simulink model "AEBMIL"  (Simulink 8.2)
settings: Solver=FixedStepDiscrete  StartTime=0.0  StopTime=126  FixedStep=0.005  RelTol=1e-3
PostLoadFcn:
  | , if any(exist('dsrtsu_mdlpostloadfcn', 'file') == [2, 3, 6]), try dsrtsu_mdlpostloadfcn('Execute', bdroot); catch fprintf('Error in PostLoadFcn (dsrtsu_mdlpostloadfcn) for model "%s":\n %s\n', bdroot, lasterr); end, end,
values from neighbouring files (symbols this model uses):
  C_TASK_5MS_S = (	C_TICK_TIME_S      	)    [hcu_local_hdr.m]
  ENUM_GEARPOSN_1ST = uint8(  1  )    [hcu_local_hdr.m]
  ENUM_GEARPOSN_R = uint8(  7  )    [hcu_local_hdr.m]
  FALSE = boolean( 0 )    [hcu_local_hdr.m]
  R_OBJ_Position = single([ii 0 0])    [GridSearch.m]
  R_OBJ_RelAccel = single([0 0 kk])    [GridSearch.m]
  R_OBJ_RelVelocity = single([0 jj 0])    [GridSearch.m]
  TRUE = boolean( 1 )    [hcu_local_hdr.m]
undefined symbols (not defined in the file or in its folder): A_OBJ, AAEB_VehSpd_kph, B_OBJ, C_OBJ, Gamma_OBJ, KAEB_AEBActiveCount_cnt, KAEB_DsblAEBAPPRateThres_pctps, KAEB_DsblAEBSteerRateThres_degps, KAEB_UseMCTTTC_flg, KAEB_VehHoldSpdThres_kph, KOBJ_KalmanFilterCalRate_s, KOBJ_UseCalObjSpd_flg, KOBJ_UseEstObjInfo_flg, KOBJ_VehAccCalRate_s, KOBJ_VehAccFltConst_s, KPTH_ObjPositionYLimit_m, MAEB_AEBTTCThres_s, MAEB_FCWTTCOffset_s, magnitude, MPTH_TurningRadius_m, Q_OBJ, slcm
libraries: simulink x49, hcu_lib x22, dspmtrx3 x3, dspinverses x1
(part 2 of 3)

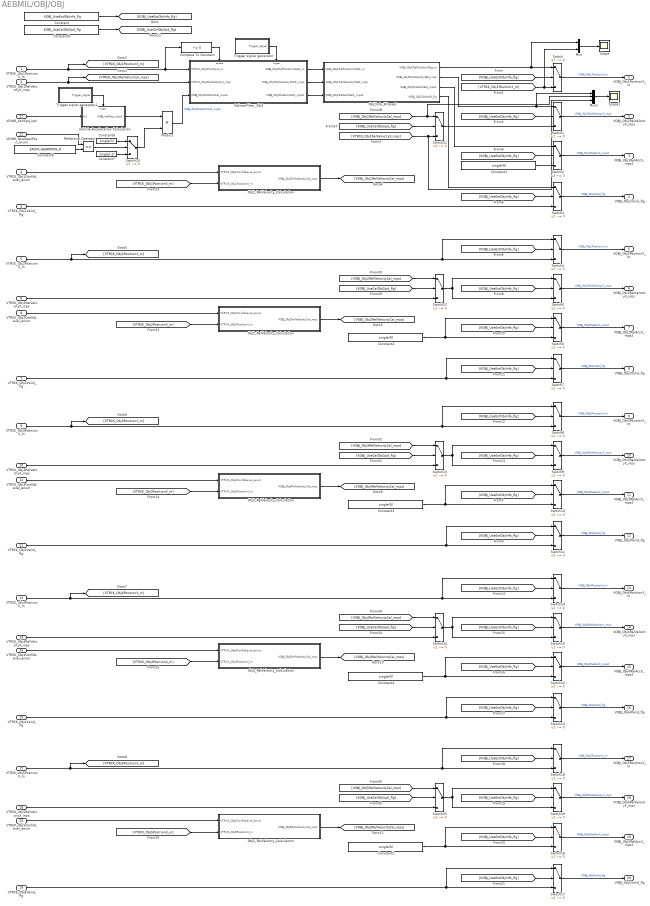
== system AEBMIL/OBJ/OBJ ==
  VTRCK_Obj1PositionX_m : Inport
  VTRCK_Obj1RelVelocityX_mps : Inport  Port=2
  VTRCK_Obj1Valid_flg : Inport  Port=3
  VTRCK_Obj1ConfidLevel_enum : Inport  Port=4
  VTRCK_Obj2PositionX_m : Inport  Port=5
  VTRCK_Obj2RelVelocityX_mps : Inport  Port=6
  VTRCK_Obj2Valid_flg : Inport  Port=7
  VTRCK_Obj2ConfidLevel_enum : Inport  Port=8
  VTRCK_Obj3PositionX_m : Inport  Port=9
  VTRCK_Obj3RelVelocityX_mps : Inport  Port=10
  VTRCK_Obj3Valid_flg : Inport  Port=11
  VTRCK_Obj3ConfidLevel_enum : Inport  Port=12
  VTRCK_Obj4PositionX_m : Inport  Port=13
  VTRCK_Obj4RelVelocityX_mps : Inport  Port=14
  VTRCK_Obj4Valid_flg : Inport  Port=15
  VTRCK_Obj4ConfidLevel_enum : Inport  Port=16
  VTRCK_Obj5PositionX_m : Inport  Port=17
  VTRCK_Obj5RelVelocityX_mps : Inport  Port=18
  VTRCK_Obj5Valid_flg : Inport  Port=19
  VTRCK_Obj5ConfidLevel_enum : Inport  Port=20
  VDINR_VehSpd_kph : Inport  Port=21
  VDINR_NowGearPosn_enum : Inport  Port=22
  Compare To Constant : simulink/Logic and Bit Operations/Compare To Constant  relop=~=  const=0  OutDataTypeStr=boolean
  Constant : Constant  Value=KOBJ_UseEstObjInfo_flg
  Constant{1..5} (5 alike) : Constant  Value=single(0)
  Constant6 : Constant  Value=single(1)
  Constant7 : Constant  Value=single(-1)
  Constant8 : Constant  Value=ENUM_GEARPOSN_R
  Constant9 : Constant  Value=KOBJ_UseCalObjSpd_flg
  KalmanFilter_Obj1 : Subsystem
  Mux : Mux  Inputs=2
  Mux1 : Mux  Inputs=3
  Obj1Info_Filtered : Subsystem
  Obj1_RelVelocity_Calculation : Subsystem
  Obj2_RelVelocity_Calculation : Subsystem
  Obj3_RelVelocity_Calculation : Subsystem
  Obj4_RelVelocity_Calculation : Subsystem
  Obj5_RelVelocity_Calculation : Subsystem
  Product : Product
  Relational Operator : RelationalOperator  Operator===  OutDataTypeStr=boolean
  Scope : Scope
  Scope1 : Scope
  Switch{,1..25} (26 alike) : Switch  Criteria=u2 ~= 0
  Trigger signal generator : Subsystem  TreatAsAtomicUnit=on
  Trigger signal generator1 : Subsystem  TreatAsAtomicUnit=on
  Vehicle Acceleration Calculation : Subsystem
  VOBJ_Obj1PositionX_m : Outport
  VOBJ_Obj1RelVelocityX_mps : Outport  Port=2
  VOBJ_Obj1RelAccX_mps2 : Outport  Port=3
  VOBJ_Obj1Valid_flg : Outport  Port=4
  VOBJ_Obj2PositionX_m : Outport  Port=5
  VOBJ_Obj2RelVelocityX_mps : Outport  Port=6
  VOBJ_Obj2RelAccX_mps2 : Outport  Port=7
  VOBJ_Obj2Valid_flg : Outport  Port=8
  VOBJ_Obj3PositionX_m : Outport  Port=9
  VOBJ_Obj3RelVelocityX_mps : Outport  Port=10
  VOBJ_Obj3RelAccX_mps2 : Outport  Port=11
  VOBJ_Obj3Valid_flg : Outport  Port=12
  VOBJ_Obj4PositionX_m : Outport  Port=13
  VOBJ_Obj4RelVelocityX_mps : Outport  Port=14
  VOBJ_Obj4RelAccX_mps2 : Outport  Port=15
  VOBJ_Obj4Valid_flg : Outport  Port=16
  VOBJ_Obj5PositionX_m : Outport  Port=17
  VOBJ_Obj5RelVelocityX_mps : Outport  Port=18
  VOBJ_Obj5RelAccX_mps2 : Outport  Port=19
  VOBJ_Obj5Valid_flg : Outport  Port=20
  wires:
  Trigger signal generator/1(Trigger_signal) -> KalmanFilter_Obj1/Trigger
  VTRCK_Obj1PositionX_m/1 -> KalmanFilter_Obj1/1(VTRCK_Obj1PositionX_m), Compare To Constant/1, [VTRCK_Obj1PositionX_m]
  VTRCK_Obj1RelVelocityX_mps/1 -> [VTRCK_Obj1RelVelocityX_mps], KalmanFilter_Obj1/2(VTRCK_Obj1RelVelocityX_mps)
  Compare To Constant/1 -> KalmanFilter_Obj1/Enable
  Trigger signal generator1/1(Trigger_signal) -> Vehicle Acceleration Calculation/Trigger
  VDINR_VehSpd_kph/1 -> Vehicle Acceleration Calculation/1(In1)
  Vehicle Acceleration Calculation/1(VOBJ_VehAcc_mps2) -> Product/1
  Product/1 -> KalmanFilter_Obj1/3(VOBJ_Obj1RelAccXCal_mps2)  "VOBJ_Obj1RelAccXCal_mps2"
  KalmanFilter_Obj1/1(VOBJ_Obj1RelPositionXKalF_m) -> Obj1Info_Filtered/1(VOBJ_Obj1RelPositionXKalF_m)
  KalmanFilter_Obj1/2(VOBJ_Obj1RelVelocityXKalF_mps) -> Obj1Info_Filtered/2(VOBJ_Obj1RelVelocityXKalF_mps)
  KalmanFilter_Obj1/3(VOBJ_Obj1RelAccXKalF_mps2) -> Obj1Info_Filtered/3(VOBJ_Obj1RelAccXKalF_mps2)
  VTRCK_Obj1Valid_flg/1 -> Switch3/3
  Constant/1 -> [KOBJ_UseEstObjInfo_flg]
  [KOBJ_UseEstObjInfo_flg] -> Switch/2
  Switch/1 -> VOBJ_Obj1PositionX_m/1  "VOBJ_Obj1PositionX_m"
  [VTRCK_Obj1PositionX_m] -> Mux/2, Switch/3
  Obj1Info_Filtered/1(VOBJ_Obj1RelPositionXEst_m) -> Mux/1, Switch/1
  [KOBJ_UseEstObjInfo_flg] -> Switch1/2
  Switch1/1 -> VOBJ_Obj1RelVelocityX_mps/1  "VOBJ_Obj1RelVelocityX_mps"
  Obj1Info_Filtered/2(VOBJ_Obj1RelVelocityXEst_mps) -> Mux1/1, Switch1/1
  [KOBJ_UseEstObjInfo_flg] -> Switch2/2
  Constant1/1 -> Switch2/3
  Obj1Info_Filtered/3(VOBJ_Obj1RelAccXEst_mps2) -> Switch2/1
  Switch2/1 -> VOBJ_Obj1RelAccX_mps2/1  "VOBJ_Obj1RelAccX_mps2"
  [KOBJ_UseEstObjInfo_flg] -> Switch3/2
  Switch3/1 -> VOBJ_Obj1Valid_flg/1  "VOBJ_Obj1Valid_flg"
  Obj1Info_Filtered/4(VOBJ_Obj1EstValid_flg) -> Switch3/1
  VTRCK_Obj2Valid_flg/1 -> Switch7/1, Switch7/3
  [KOBJ_UseEstObjInfo_flg] -> Switch4/2
  Switch4/1 -> VOBJ_Obj2PositionX_m/1  "VOBJ_Obj2PositionX_m"
  VTRCK_Obj2PositionX_m/1 -> [VTRCK_Obj2PositionX_m], Switch4/1, Switch4/3
  [KOBJ_UseEstObjInfo_flg] -> Switch5/2
  Switch5/1 -> VOBJ_Obj2RelVelocityX_mps/1  "VOBJ_Obj2RelVelocityX_mps"
  [KOBJ_UseEstObjInfo_flg] -> Switch6/2
  Constant2/1 -> Switch6/1, Switch6/3
  Switch6/1 -> VOBJ_Obj2RelAccX_mps2/1  "VOBJ_Obj2RelAccX_mps2"
  [KOBJ_UseEstObjInfo_flg] -> Switch7/2
  Switch7/1 -> VOBJ_Obj2Valid_flg/1  "VOBJ_Obj2Valid_flg"
  VTRCK_Obj3Valid_flg/1 -> Switch11/3, Switch11/1
  [KOBJ_UseEstObjInfo_flg] -> Switch8/2
  Switch8/1 -> VOBJ_Obj3PositionX_m/1  "VOBJ_Obj3PositionX_m"
  VTRCK_Obj3PositionX_m/1 -> [VTRCK_Obj3PositionX_m], Switch8/3, Switch8/1
  [KOBJ_UseEstObjInfo_flg] -> Switch9/2
  Switch9/1 -> VOBJ_Obj3RelVelocityX_mps/1  "VOBJ_Obj3RelVelocityX_mps"
  VTRCK_Obj3RelVelocityX_mps/1 -> Switch23/3
  [KOBJ_UseEstObjInfo_flg] -> Switch10/2
  Constant3/1 -> Switch10/3, Switch10/1
  Switch10/1 -> VOBJ_Obj3RelAccX_mps2/1  "VOBJ_Obj3RelAccX_mps2"
  [KOBJ_UseEstObjInfo_flg] -> Switch11/2
  Switch11/1 -> VOBJ_Obj3Valid_flg/1  "VOBJ_Obj3Valid_flg"
  VTRCK_Obj4Valid_flg/1 -> Switch13/1, Switch13/3
  [KOBJ_UseEstObjInfo_flg] -> Switch14/2
  Switch14/1 -> VOBJ_Obj4PositionX_m/1  "VOBJ_Obj4PositionX_m"
  VTRCK_Obj4PositionX_m/1 -> [VTRCK_Obj4PositionX_m], Switch14/1, Switch14/3
  [KOBJ_UseEstObjInfo_flg] -> Switch15/2
  Switch15/1 -> VOBJ_Obj4RelVelocityX_mps/1  "VOBJ_Obj4RelVelocityX_mps"
  VTRCK_Obj4RelVelocityX_mps/1 -> Switch24/3
  [KOBJ_UseEstObjInfo_flg] -> Switch12/2
  Constant4/1 -> Switch12/1, Switch12/3
  Switch12/1 -> VOBJ_Obj4RelAccX_mps2/1  "VOBJ_Obj4RelAccX_mps2"
  [KOBJ_UseEstObjInfo_flg] -> Switch13/2
  Switch13/1 -> VOBJ_Obj4Valid_flg/1  "VOBJ_Obj4Valid_flg"
  VTRCK_Obj5Valid_flg/1 -> Switch17/3, Switch17/1
  [KOBJ_UseEstObjInfo_flg] -> Switch18/2
  Switch18/1 -> VOBJ_Obj5PositionX_m/1  "VOBJ_Obj5PositionX_m"
  VTRCK_Obj5PositionX_m/1 -> [VTRCK_Obj5PositionX_m], Switch18/3, Switch18/1
  [KOBJ_UseEstObjInfo_flg] -> Switch19/2
  Switch19/1 -> VOBJ_Obj5RelVelocityX_mps/1  "VOBJ_Obj5RelVelocityX_mps"
  VTRCK_Obj5RelVelocityX_mps/1 -> Switch25/3
  [KOBJ_UseEstObjInfo_flg] -> Switch16/2
  Constant5/1 -> Switch16/3, Switch16/1
  Switch16/1 -> VOBJ_Obj5RelAccX_mps2/1  "VOBJ_Obj5RelAccX_mps2"
  [KOBJ_UseEstObjInfo_flg] -> Switch17/2
  Switch17/1 -> VOBJ_Obj5Valid_flg/1  "VOBJ_Obj5Valid_flg"
  VDINR_NowGearPosn_enum/1 -> Relational Operator/1
  Constant8/1 -> Relational Operator/2
  Relational Operator/1 -> Switch20/2
  Constant6/1 -> Switch20/1
  Constant7/1 -> Switch20/3
  Switch20/1 -> Product/2
  VTRCK_Obj5ConfidLevel_enum/1 -> Obj5_RelVelocity_Calculation/1(VTRCK_Obj5ConfidLevel_enum)
  [VTRCK_Obj5PositionX_m] -> Obj5_RelVelocity_Calculation/2(VTRCK_Obj5PositionX_m)
  Obj5_RelVelocity_Calculation/1(VOBJ_Obj5RelVelocityCal_mps) -> [VOBJ_Obj5RelVelocityCal_mps]
  VTRCK_Obj4ConfidLevel_enum/1 -> Obj4_RelVelocity_Calculation/1(VTRCK_Obj4ConfidLevel_enum)
  [VTRCK_Obj4PositionX_m] -> Obj4_RelVelocity_Calculation/2(VTRCK_Obj4PositionX_m)
  Obj4_RelVelocity_Calculation/1(VOBJ_Obj4RelVelocityCal_mps) -> [VOBJ_Obj4RelVelocityCal_mps]
  VTRCK_Obj3ConfidLevel_enum/1 -> Obj3_RelVelocity_Calculation/1(VTRCK_Obj3ConfidLevel_enum)
  [VTRCK_Obj3PositionX_m] -> Obj3_RelVelocity_Calculation/2(VTRCK_Obj3PositionX_m)
  Obj3_RelVelocity_Calculation/1(VOBJ_Obj3RelVelocityCal_mps) -> [VOBJ_Obj3RelVelocityCal_mps]
  VTRCK_Obj2ConfidLevel_enum/1 -> Obj2_RelVelocity_Calculation/1(VTRCK_Obj2ConfidLevel_enum)
  [VTRCK_Obj2PositionX_m] -> Obj2_RelVelocity_Calculation/2(VTRCK_Obj2PositionX_m)
  Obj2_RelVelocity_Calculation/1(VOBJ_Obj2RelVelocityCal_mps) -> [VOBJ_Obj2RelVelocityCal_mps]
  VTRCK_Obj1ConfidLevel_enum/1 -> Obj1_RelVelocity_Calculation/1(VTRCK_Obj1ConfidLevel_enum)
  [VTRCK_Obj1PositionX_m] -> Obj1_RelVelocity_Calculation/2(VTRCK_Obj1PositionX_m)
  Obj1_RelVelocity_Calculation/1(VOBJ_Obj1RelVelocityCal_mps) -> [VOBJ_Obj1RelVelocityCal_mps]
  Constant9/1 -> [KOBJ_UseCalObjSpd_flg]
  [KOBJ_UseCalObjSpd_flg] -> Switch21/2
  [VOBJ_Obj1RelVelocityCal_mps] -> Mux1/2, Switch21/1
  [VTRCK_Obj1RelVelocityX_mps] -> Mux1/3, Switch21/3
  Switch21/1 -> Switch1/3
  [KOBJ_UseCalObjSpd_flg] -> Switch22/2
  [VOBJ_Obj2RelVelocityCal_mps] -> Switch22/1
  VTRCK_Obj2RelVelocityX_mps/1 -> Switch22/3
  Switch22/1 -> Switch5/3, Switch5/1
  [KOBJ_UseCalObjSpd_flg] -> Switch23/2
  [VOBJ_Obj3RelVelocityCal_mps] -> Switch23/1
  Switch23/1 -> Switch9/1, Switch9/3
  [KOBJ_UseCalObjSpd_flg] -> Switch24/2
  [VOBJ_Obj4RelVelocityCal_mps] -> Switch24/1
  Switch24/1 -> Switch15/1, Switch15/3
  [KOBJ_UseCalObjSpd_flg] -> Switch25/2
  [VOBJ_Obj5RelVelocityCal_mps] -> Switch25/1
  Switch25/1 -> Switch19/1, Switch19/3
  Mux/1 -> Scope/1
  Mux1/1 -> Scope1/1

== system AEBMIL/OBJ/model_info ==
  EmptySubsystem : Subsystem

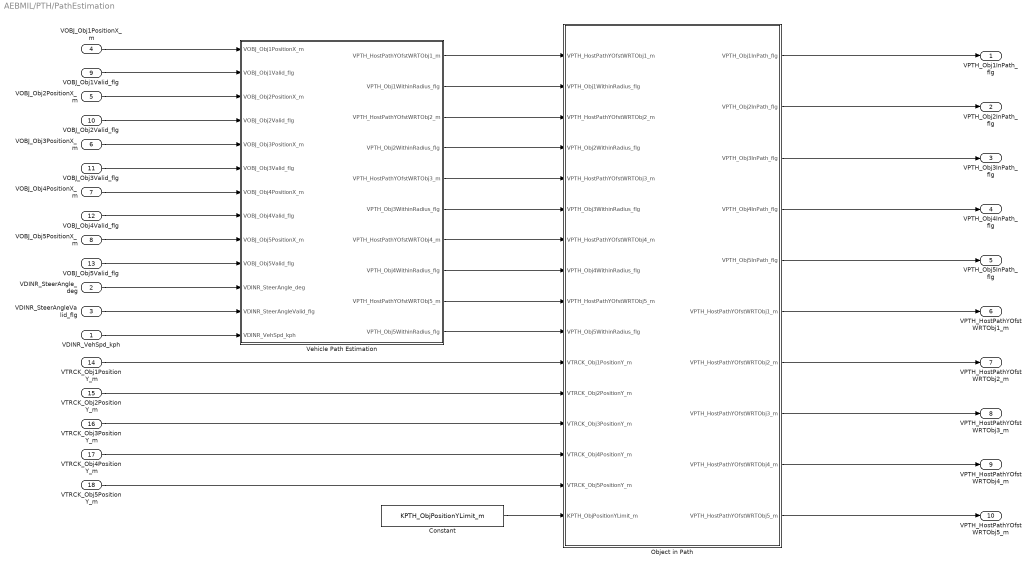
== system AEBMIL/PTH/PathEstimation ==
  VDINR_VehSpd_kph : Inport
  VDINR_SteerAngle_deg : Inport  Port=2
  VDINR_SteerAngleValid_flg : Inport  Port=3
  VOBJ_Obj1PositionX_m : Inport  Port=4
  VOBJ_Obj2PositionX_m : Inport  Port=5
  VOBJ_Obj3PositionX_m : Inport  Port=6
  VOBJ_Obj4PositionX_m : Inport  Port=7
  VOBJ_Obj5PositionX_m : Inport  Port=8
  VOBJ_Obj1Valid_flg : Inport  Port=9
  VOBJ_Obj2Valid_flg : Inport  Port=10
  VOBJ_Obj3Valid_flg : Inport  Port=11
  VOBJ_Obj4Valid_flg : Inport  Port=12
  VOBJ_Obj5Valid_flg : Inport  Port=13
  VTRCK_Obj1PositionY_m : Inport  Port=14
  VTRCK_Obj2PositionY_m : Inport  Port=15
  VTRCK_Obj3PositionY_m : Inport  Port=16
  VTRCK_Obj4PositionY_m : Inport  Port=17
  VTRCK_Obj5PositionY_m : Inport  Port=18
  Constant : Constant  Value=KPTH_ObjPositionYLimit_m
  Object in Path : Subsystem
  Vehicle Path Estimation : Subsystem
  VPTH_Obj1InPath_flg : Outport
  VPTH_Obj2InPath_flg : Outport  Port=2
  VPTH_Obj3InPath_flg : Outport  Port=3
  VPTH_Obj4InPath_flg : Outport  Port=4
  VPTH_Obj5InPath_flg : Outport  Port=5
  VPTH_HostPathYOfstWRTObj1_m : Outport  Port=6
  VPTH_HostPathYOfstWRTObj2_m : Outport  Port=7
  VPTH_HostPathYOfstWRTObj3_m : Outport  Port=8
  VPTH_HostPathYOfstWRTObj4_m : Outport  Port=9
  VPTH_HostPathYOfstWRTObj5_m : Outport  Port=10
  wires:
  Object in Path/10("VPTH_HostPathYOfstWRTObj5_m ") -> VPTH_HostPathYOfstWRTObj5_m/1
  Object in Path/9("VPTH_HostPathYOfstWRTObj4_m ") -> VPTH_HostPathYOfstWRTObj4_m/1
  Object in Path/8("VPTH_HostPathYOfstWRTObj3_m ") -> VPTH_HostPathYOfstWRTObj3_m/1
  Object in Path/7("VPTH_HostPathYOfstWRTObj2_m ") -> VPTH_HostPathYOfstWRTObj2_m/1
  Object in Path/6("VPTH_HostPathYOfstWRTObj1_m ") -> VPTH_HostPathYOfstWRTObj1_m/1
  VOBJ_Obj5Valid_flg/1 -> Vehicle Path Estimation/10(VOBJ_Obj5Valid_flg)
  VOBJ_Obj4Valid_flg/1 -> Vehicle Path Estimation/8(VOBJ_Obj4Valid_flg)
  VOBJ_Obj3Valid_flg/1 -> Vehicle Path Estimation/6(VOBJ_Obj3Valid_flg)
  VOBJ_Obj2Valid_flg/1 -> Vehicle Path Estimation/4(VOBJ_Obj2Valid_flg)
  VOBJ_Obj1Valid_flg/1 -> Vehicle Path Estimation/2(VOBJ_Obj1Valid_flg)
  Object in Path/5(VPTH_Obj5InPath_flg) -> VPTH_Obj5InPath_flg/1
  Object in Path/4(VPTH_Obj4InPath_flg) -> VPTH_Obj4InPath_flg/1
  Object in Path/3(VPTH_Obj3InPath_flg) -> VPTH_Obj3InPath_flg/1
  Object in Path/2(VPTH_Obj2InPath_flg) -> VPTH_Obj2InPath_flg/1
  VTRCK_Obj2PositionY_m/1 -> Object in Path/12(VTRCK_Obj2PositionY_m)
  VTRCK_Obj3PositionY_m/1 -> Object in Path/13(VTRCK_Obj3PositionY_m)
  VTRCK_Obj5PositionY_m/1 -> Object in Path/15(VTRCK_Obj5PositionY_m)
  VTRCK_Obj4PositionY_m/1 -> Object in Path/14(VTRCK_Obj4PositionY_m)
  Vehicle Path Estimation/10(VPTH_Obj5WithinRadius_flg) -> Object in Path/10(VPTH_Obj5WithinRadius_flg)
  Vehicle Path Estimation/9(VPTH_HostPathYOfstWRTObj5_m) -> Object in Path/9(VPTH_HostPathYOfstWRTObj5_m)
  Vehicle Path Estimation/8(VPTH_Obj4WithinRadius_flg) -> Object in Path/8(VPTH_Obj4WithinRadius_flg)
  Vehicle Path Estimation/7(VPTH_HostPathYOfstWRTObj4_m) -> Object in Path/7(VPTH_HostPathYOfstWRTObj4_m)
  Vehicle Path Estimation/6(VPTH_Obj3WithinRadius_flg) -> Object in Path/6(VPTH_Obj3WithinRadius_flg)
  Vehicle Path Estimation/5(VPTH_HostPathYOfstWRTObj3_m) -> Object in Path/5(VPTH_HostPathYOfstWRTObj3_m)
  Vehicle Path Estimation/4(VPTH_Obj2WithinRadius_flg) -> Object in Path/4(VPTH_Obj2WithinRadius_flg)
  Vehicle Path Estimation/3(VPTH_HostPathYOfstWRTObj2_m) -> Object in Path/3(VPTH_HostPathYOfstWRTObj2_m)
  VOBJ_Obj5PositionX_m/1 -> Vehicle Path Estimation/9(VOBJ_Obj5PositionX_m)
  VOBJ_Obj4PositionX_m/1 -> Vehicle Path Estimation/7(VOBJ_Obj4PositionX_m)
  VOBJ_Obj3PositionX_m/1 -> Vehicle Path Estimation/5(VOBJ_Obj3PositionX_m)
  VOBJ_Obj2PositionX_m/1 -> Vehicle Path Estimation/3(VOBJ_Obj2PositionX_m)
  VDINR_SteerAngleValid_flg/1 -> Vehicle Path Estimation/12(VDINR_SteerAngleValid_flg)
  VDINR_VehSpd_kph/1 -> Vehicle Path Estimation/13(VDINR_VehSpd_kph)
  VOBJ_Obj1PositionX_m/1 -> Vehicle Path Estimation/1(VOBJ_Obj1PositionX_m)
  VDINR_SteerAngle_deg/1 -> Vehicle Path Estimation/11(VDINR_SteerAngle_deg)
  VTRCK_Obj1PositionY_m/1 -> Object in Path/11(VTRCK_Obj1PositionY_m)
  Constant/1 -> Object in Path/16(KPTH_ObjPositionYLimit_m)
  Vehicle Path Estimation/1(VPTH_HostPathYOfstWRTObj1_m) -> Object in Path/1(VPTH_HostPathYOfstWRTObj1_m)
  Object in Path/1(VPTH_Obj1InPath_flg) -> VPTH_Obj1InPath_flg/1
  Vehicle Path Estimation/2(VPTH_Obj1WithinRadius_flg) -> Object in Path/2(VPTH_Obj1WithinRadius_flg)

== system AEBMIL/PTH/model_info ==
  EmptySubsystem : Subsystem

== system AEBMIL/TTC/MCT_TTC_Calculation ==
  VMCT_MCTRelPositionX_m : Inport
  VMCT_MCTRelVelocityX_mps : Inport  Port=2
  VMCT_MCTValid_flg : Inport  Port=3
  VMCT_MCTInPath_flg : Inport  Port=4
  Constant1 : Constant  Value=-99  OutDataTypeStr=single
  Data Type Conversion : DataTypeConversion  OutDataTypeStr=single
  Data Type Conversion1 : DataTypeConversion  OutDataTypeStr=single
  Gain4 : Gain  Gain=-1
  Product : Product  Inputs=3  RndMeth=Zero
  divide : hcu_lib/divide
  VTTC_MCTTTC_s : Outport
  wires:
  Data Type Conversion1/1 -> Product/3
  Data Type Conversion/1 -> Product/2
  VMCT_MCTInPath_flg/1 -> Data Type Conversion1/1
  VMCT_MCTRelVelocityX_mps/1 -> Product/1
  VMCT_MCTRelPositionX_m/1 -> divide/1
  Product/1 -> divide/2
  VMCT_MCTValid_flg/1 -> Data Type Conversion/1
  Constant1/1 -> divide/3
  divide/1 -> Gain4/1
  Gain4/1 -> VTTC_MCTTTC_s/1  "VTTC_MCTTTC_s"

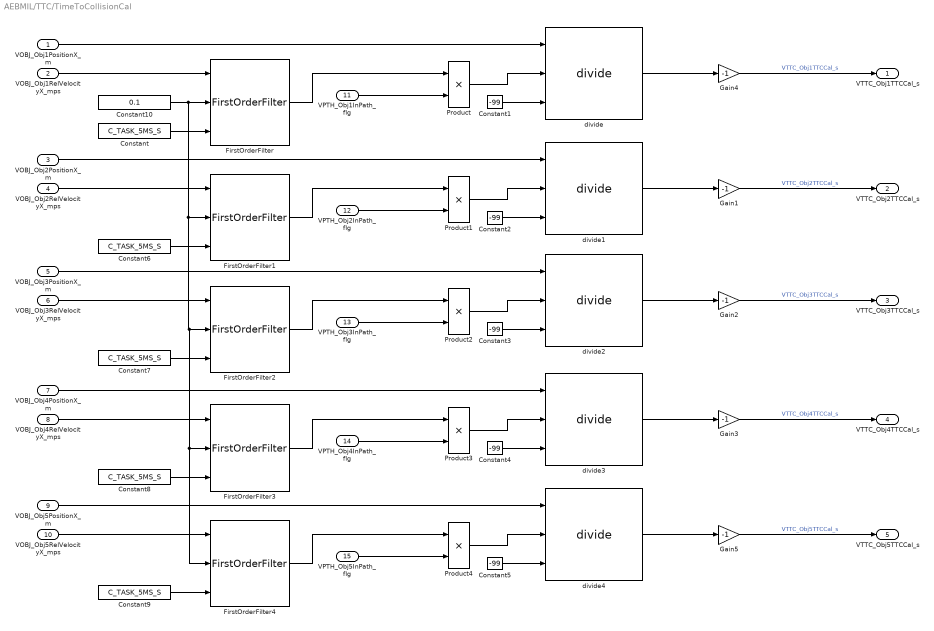
== system AEBMIL/TTC/TimeToCollisionCal ==
  VOBJ_Obj1PositionX_m : Inport
  VOBJ_Obj1RelVelocityX_mps : Inport  Port=2
  VOBJ_Obj2PositionX_m : Inport  Port=3
  VOBJ_Obj2RelVelocityX_mps : Inport  Port=4
  VOBJ_Obj3PositionX_m : Inport  Port=5
  VOBJ_Obj3RelVelocityX_mps : Inport  Port=6
  VOBJ_Obj4PositionX_m : Inport  Port=7
  VOBJ_Obj4RelVelocityX_mps : Inport  Port=8
  VOBJ_Obj5PositionX_m : Inport  Port=9
  VOBJ_Obj5RelVelocityX_mps : Inport  Port=10
  VPTH_Obj1InPath_flg : Inport  Port=11
  VPTH_Obj2InPath_flg : Inport  Port=12
  VPTH_Obj3InPath_flg : Inport  Port=13
  VPTH_Obj4InPath_flg : Inport  Port=14
  VPTH_Obj5InPath_flg : Inport  Port=15
  Constant{,6..9} (5 alike) : Constant  Value=C_TASK_5MS_S
  Constant{1..5} (5 alike) : Constant  Value=-99  OutDataTypeStr=single
  Constant10 : Constant  Value=0.1  OutDataTypeStr=single
  FirstOrderFilter{,1..4} (5 alike) : hcu_lib/FirstOrderFilter
  Gain{1..5} (5 alike) : Gain  Gain=-1
  Product{,1..4} (5 alike) : Product  RndMeth=Zero
  divide{,1..4} (5 alike) : hcu_lib/divide
  VTTC_Obj1TTCCal_s : Outport
  VTTC_Obj2TTCCal_s : Outport  Port=2
  VTTC_Obj3TTCCal_s : Outport  Port=3
  VTTC_Obj4TTCCal_s : Outport  Port=4
  VTTC_Obj5TTCCal_s : Outport  Port=5
  wires:
  FirstOrderFilter4/1 -> Product4/1
  FirstOrderFilter3/1 -> Product3/1
  FirstOrderFilter2/1 -> Product2/1
  FirstOrderFilter1/1 -> Product1/1
  FirstOrderFilter/1 -> Product/1
  divide4/1 -> Gain5/1
  divide3/1 -> Gain3/1
  divide2/1 -> Gain2/1
  divide1/1 -> Gain1/1
  divide/1 -> Gain4/1
  Constant10/1 -> FirstOrderFilter/2, FirstOrderFilter1/2, FirstOrderFilter2/2, FirstOrderFilter3/2, FirstOrderFilter4/2
  Constant9/1 -> FirstOrderFilter4/3
  Constant8/1 -> FirstOrderFilter3/3
  Constant7/1 -> FirstOrderFilter2/3
  Constant6/1 -> FirstOrderFilter1/3
  Constant/1 -> FirstOrderFilter/3
  VOBJ_Obj5PositionX_m/1 -> divide4/1
  Gain5/1 -> VTTC_Obj5TTCCal_s/1  "VTTC_Obj5TTCCal_s"
  VOBJ_Obj5RelVelocityX_mps/1 -> FirstOrderFilter4/1
  Constant5/1 -> divide4/3
  VPTH_Obj5InPath_flg/1 -> Product4/2
  Product4/1 -> divide4/2
  VOBJ_Obj4PositionX_m/1 -> divide3/1
  Gain3/1 -> VTTC_Obj4TTCCal_s/1  "VTTC_Obj4TTCCal_s"
  VOBJ_Obj4RelVelocityX_mps/1 -> FirstOrderFilter3/1
  Constant4/1 -> divide3/3
  VPTH_Obj4InPath_flg/1 -> Product3/2
  Product3/1 -> divide3/2
  VOBJ_Obj3PositionX_m/1 -> divide2/1
  Gain2/1 -> VTTC_Obj3TTCCal_s/1  "VTTC_Obj3TTCCal_s"
  VOBJ_Obj3RelVelocityX_mps/1 -> FirstOrderFilter2/1
  Constant3/1 -> divide2/3
  VPTH_Obj3InPath_flg/1 -> Product2/2
  Product2/1 -> divide2/2
  VOBJ_Obj2PositionX_m/1 -> divide1/1
  Gain1/1 -> VTTC_Obj2TTCCal_s/1  "VTTC_Obj2TTCCal_s"
  VOBJ_Obj2RelVelocityX_mps/1 -> FirstOrderFilter1/1
  Constant2/1 -> divide1/3
  VPTH_Obj2InPath_flg/1 -> Product1/2
  Product1/1 -> divide1/2
  VOBJ_Obj1PositionX_m/1 -> divide/1
  Gain4/1 -> VTTC_Obj1TTCCal_s/1  "VTTC_Obj1TTCCal_s"
  VOBJ_Obj1RelVelocityX_mps/1 -> FirstOrderFilter/1
  Constant1/1 -> divide/3
  VPTH_Obj1InPath_flg/1 -> Product/2
  Product/1 -> divide/2

== system AEBMIL/TTC/model_info ==
  EmptySubsystem : Subsystem

== system AEBMIL/AEB/AEB/AEB Determination ==
  VAEB_DriverDisable_flg : Inport
  VAEB_DriverDisableLatch_flg : Inport  Port=2
  VDINR_SeatBeltNOTFasten_flg : Inport  Port=3
  VDINR_VehSpd_kph : Inport  Port=4
  VTTC_MCTTTC_s : Inport  Port=5
  VTTC_Obj1TTCCal_s : Inport  Port=6
  AEB_Brain : Subsystem
  LookAhead Distance Gain Lookup1 : Lookup  InputValues=AAEB_VehSpd_kph  Table=MAEB_FCWTTCOffset_s  LookUpMeth=Interpolation-Use End Values
      settings: AttributesFormatString=%<InputValues>\n%<Table>
  LookAhead Distance Gain Lookup2 : Lookup  InputValues=AAEB_VehSpd_kph  Table=MAEB_AEBTTCThres_s  LookUpMeth=Interpolation-Use End Values
      settings: AttributesFormatString=%<InputValues>\n%<Table>
  Terminator : Terminator
  VAEB_AEBActive_flg : Outport
  VAEB_FCWActive_flg : Outport  Port=2
  VAEB_ForcedIdle_flg : Outport  Port=3
  VAEB_PreFillReq_flg : Outport  Port=4
  VAEB_VehHoldReq_flg : Outport  Port=5
  wires:
  VTTC_Obj1TTCCal_s/1 -> AEB_Brain/7(VTTC_Obj1TTCCal_s)
  AEB_Brain/5(VAEB_VehHoldReq_flg) -> VAEB_VehHoldReq_flg/1
  AEB_Brain/4(VAEB_PreFillReq_flg) -> VAEB_PreFillReq_flg/1
  AEB_Brain/3(VAEB_ForcedIdle_flg) -> VAEB_ForcedIdle_flg/1
  AEB_Brain/2(VAEB_FCWActive_flg) -> VAEB_FCWActive_flg/1
  VTTC_MCTTTC_s/1 -> AEB_Brain/6(VTTC_MCTTTC_s)
  VDINR_SeatBeltNOTFasten_flg/1 -> AEB_Brain/5(VDINR_SeatBeltNOTFasten_flg)
  VAEB_DriverDisableLatch_flg/1 -> Terminator/1
  LookAhead Distance Gain Lookup1/1 -> AEB_Brain/2(FCWTTCOffset)
  AEB_Brain/1(VAEB_AEBActive_flg) -> VAEB_AEBActive_flg/1
  VDINR_VehSpd_kph/1 -> LookAhead Distance Gain Lookup2/1, LookAhead Distance Gain Lookup1/1, AEB_Brain/3(VDINR_VehSpd_kph)
  LookAhead Distance Gain Lookup2/1 -> AEB_Brain/1(AEBTTCThres)
  VAEB_DriverDisable_flg/1 -> AEB_Brain/4(VAEB_DriverDisable_flg)

== system AEBMIL/AEB/AEB/Driver Disable ==
  VDINR_SteerAngle_deg : Inport
  VDINR_SteerAngleValid_flg : Inport  Port=2
  VDINR_HWAccelPedalPosn_pct : Inport  Port=3
  VDINR_HWAccelPedalPosnValid_flg : Inport  Port=4
  VAEB_AEBActive_flg : Inport  Port=5
  APPRateCalculation : Subsystem  TreatAsAtomicUnit=on
  Abs1 : Abs
  Constant1 : Constant  Value=KAEB_DsblAEBAPPRateThres_pctps
  Constant2 : Constant  Value=KAEB_DsblAEBSteerRateThres_degps
  Function-Call Generator : Stateflow chart  TreatAsAtomicUnit=on
  Logical Operator : Logic  Operator=NOT  AllPortsSameDT=off  OutDataTypeStr=boolean
  Logical Operator8 : Logic  Operator=OR  AllPortsSameDT=off  OutDataTypeStr=boolean
  Relational Operator1 : RelationalOperator  OutDataTypeStr=boolean
  Relational Operator3 : RelationalOperator  OutDataTypeStr=boolean
  SR-Latch : hcu_lib/SR-Latch
  SteeringRateCalculation : Subsystem  TreatAsAtomicUnit=on
  VAEB_DriverDisable_flg : Outport
  VAEB_DriverDisableLatch_flg : Outport  Port=2
  wires:
  Logical Operator/1 -> SR-Latch/2
  SR-Latch/1 -> VAEB_DriverDisableLatch_flg/1  "VAEB_DriverDisableLatch_flg"
  Logical Operator8/1 -> SR-Latch/1, VAEB_DriverDisable_flg/1  "VAEB_DriverDisable_flg"
  VAEB_AEBActive_flg/1 -> Logical Operator/1
  Relational Operator1/1 -> Logical Operator8/2
  APPRateCalculation/1(VAEB_APPMovingRate_pctps) -> Relational Operator1/1
  Abs1/1 -> Relational Operator3/1
  Constant1/1 -> Relational Operator1/2
  VDINR_HWAccelPedalPosnValid_flg/1 -> APPRateCalculation/2(VDINR_HWAccelPedalPosnValid_flg)
  VDINR_HWAccelPedalPosn_pct/1 -> APPRateCalculation/1(VDINR_HWAccelPedalPosn_pct)
  SteeringRateCalculation/1(VAEB_SteeringRate_degps) -> Abs1/1
  VDINR_SteerAngleValid_flg/1 -> SteeringRateCalculation/2(VDINR_SteerAngleValid_flg)
  [trig_APPINTEND] -> APPRateCalculation/Trigger
  [trig_STEERINTEND] -> SteeringRateCalculation/Trigger
  Function-Call Generator/2(trig_APPINTEND()) -> [trig_APPINTEND]
  Function-Call Generator/1(trig_STEERINTEND()) -> [trig_STEERINTEND]
  VDINR_SteerAngle_deg/1 -> SteeringRateCalculation/1(VDINR_SteerAngle_deg)
  Relational Operator3/1 -> Logical Operator8/1
  Constant2/1 -> Relational Operator3/2

== system AEBMIL/AEB/model_info/EmptySubsystem ==

== system AEBMIL/MCT/MCT/Switch Case Action Subsystem ==
  Action Port : ActionPort  ActionType=then
  Constant : Constant  Value=uint8(1)
  Out1 : Outport
  wires:
  Constant/1 -> Out1/1

== system AEBMIL/MCT/MCT/Switch Case Action Subsystem1 ==
  Action Port : ActionPort  ActionType=elseif
  Constant : Constant  Value=uint8(2)
  Out1 : Outport
  wires:
  Constant/1 -> Out1/1

== system AEBMIL/MCT/MCT/Switch Case Action Subsystem2 ==
  Action Port : ActionPort  ActionType=elseif
  Constant : Constant  Value=uint8(3)
  Out1 : Outport
  wires:
  Constant/1 -> Out1/1

== system AEBMIL/MCT/MCT/Switch Case Action Subsystem3 ==
  Action Port : ActionPort  ActionType=elseif
  Constant : Constant  Value=uint8(4)
  Out1 : Outport
  wires:
  Constant/1 -> Out1/1

== system AEBMIL/MCT/MCT/Switch Case Action Subsystem4 ==
  Action Port : ActionPort  ActionType=elseif
  Constant : Constant  Value=uint8(5)
  Out1 : Outport
  wires:
  Constant/1 -> Out1/1

== system AEBMIL/MCT/MCT/Switch Case Action Subsystem5 ==
  Action Port : ActionPort  ActionType=else
  Constant : Constant  Value=uint8(0)
  Out1 : Outport
  wires:
  Constant/1 -> Out1/1

== system AEBMIL/MCT/model_info/EmptySubsystem ==

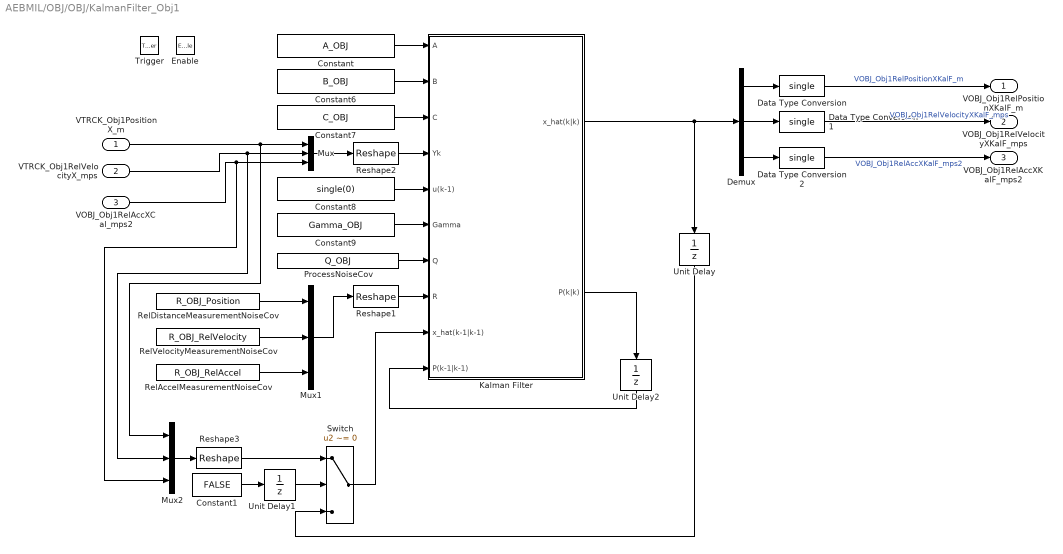
== system AEBMIL/OBJ/OBJ/KalmanFilter_Obj1 ==
  VTRCK_Obj1PositionX_m : Inport
  VTRCK_Obj1RelVelocityX_mps : Inport  Port=2
  VOBJ_Obj1RelAccXCal_mps2 : Inport  Port=3
  Enable : EnablePort  StatesWhenEnabling=reset
  Trigger : TriggerPort  PortDimensions=1
  Constant : Constant  Value=A_OBJ
  Constant1 : Constant  Value=FALSE
  Constant6 : Constant  Value=B_OBJ
  Constant7 : Constant  Value=C_OBJ
  Constant8 : Constant  Value=single(0)
  Constant9 : Constant  Value=Gamma_OBJ
  Data Type Conversion : DataTypeConversion  OutDataTypeStr=single
  Data Type Conversion1 : DataTypeConversion  OutDataTypeStr=single
  Data Type Conversion2 : DataTypeConversion  OutDataTypeStr=single
  Demux : Demux  Outputs=3
  Kalman Filter : Subsystem
  Mux : Mux  Inputs=3
  Mux1 : Mux  Inputs=3
  Mux2 : Mux  Inputs=3
  ProcessNoiseCov : Constant  Value=Q_OBJ
  RelAccelMeasurementNoiseCov : Constant  Value=R_OBJ_RelAccel  OutDataTypeStr=single
  RelDistanceMeasurementNoiseCov : Constant  Value=R_OBJ_Position  OutDataTypeStr=single
  RelVelocityMeasurementNoiseCov : Constant  Value=R_OBJ_RelVelocity  OutDataTypeStr=single
  Reshape1 : Reshape  OutputDimensionality=Customize  OutputDimensions=[3,3]
  Reshape2 : Reshape  OutputDimensionality=Customize  OutputDimensions=[3,1]
  Reshape3 : Reshape  OutputDimensionality=Customize  OutputDimensions=[3,1]
  Switch : Switch  Criteria=u2 ~= 0
  Unit Delay : UnitDelay  InitialCondition=single([0;0;0])  SampleTime=-1
  Unit Delay1 : UnitDelay  InitialCondition=TRUE  SampleTime=-1
  Unit Delay2 : UnitDelay  InitialCondition=single(eye(3,3))  SampleTime=-1
  VOBJ_Obj1RelPositionXKalF_m : Outport  OutputWhenDisabled=reset  InitialOutput=[0]
  VOBJ_Obj1RelVelocityXKalF_mps : Outport  Port=2  OutputWhenDisabled=reset  InitialOutput=[0]
  VOBJ_Obj1RelAccXKalF_mps2 : Outport  Port=3  OutputWhenDisabled=reset  InitialOutput=[0]
  wires:
  Data Type Conversion2/1 -> VOBJ_Obj1RelAccXKalF_mps2/1  "VOBJ_Obj1RelAccXKalF_mps2"
  Data Type Conversion1/1 -> VOBJ_Obj1RelVelocityXKalF_mps/1  "VOBJ_Obj1RelVelocityXKalF_mps"
  Data Type Conversion/1 -> VOBJ_Obj1RelPositionXKalF_m/1  "VOBJ_Obj1RelPositionXKalF_m"
  Kalman Filter/2(P(k|k)) -> Unit Delay2/1
  Unit Delay2/1 -> Kalman Filter/10(P(k-1|k-1))
  Kalman Filter/1(x_hat(k|k)) -> Unit Delay/1, Demux/1
  Unit Delay/1 -> Switch/3
  Constant9/1 -> Kalman Filter/6(Gamma)
  ProcessNoiseCov/1 -> Kalman Filter/7(Q)
  Mux1/1 -> Reshape1/1
  Reshape2/1 -> Kalman Filter/4(Yk)
  Mux/1 -> Reshape2/1
  Constant8/1 -> Kalman Filter/5(u(k-1))
  Constant/1 -> Kalman Filter/1(A)
  Constant6/1 -> Kalman Filter/2(B)
  Constant7/1 -> Kalman Filter/3(C)
  RelDistanceMeasurementNoiseCov/1 -> Mux1/1
  RelVelocityMeasurementNoiseCov/1 -> Mux1/2
  Reshape1/1 -> Kalman Filter/8(R)
  VTRCK_Obj1RelVelocityX_mps/1 -> Mux2/2, Mux/2
  VTRCK_Obj1PositionX_m/1 -> Mux2/1, Mux/1
  Demux/2 -> Data Type Conversion1/1
  Demux/1 -> Data Type Conversion/1
  Demux/3 -> Data Type Conversion2/1
  Constant1/1 -> Unit Delay1/1
  Unit Delay1/1 -> Switch/2
  VOBJ_Obj1RelAccXCal_mps2/1 -> Mux2/3, Mux/3
  Mux2/1 -> Reshape3/1
  Reshape3/1 -> Switch/1
  Switch/1 -> Kalman Filter/9(x_hat(k-1|k-1))
  RelAccelMeasurementNoiseCov/1 -> Mux1/3

== system AEBMIL/OBJ/OBJ/Obj1Info_Filtered ==
  VOBJ_Obj1RelPositionXKalF_m : Inport
  VOBJ_Obj1RelVelocityXKalF_mps : Inport  Port=2
  VOBJ_Obj1RelAccXKalF_mps2 : Inport  Port=3
  Compare To Zero : simulink/Logic and Bit Operations/Compare To Zero  relop=~=  OutDataTypeStr=boolean
  Constant : Constant  Value=single(0)
  Constant1 : Constant  Value=single(0)
  Constant2 : Constant  Value=single(0)
  Switch : Switch  Criteria=u2 ~= 0
  Switch1 : Switch  Criteria=u2 ~= 0
  Switch2 : Switch  Criteria=u2 ~= 0
  VOBJ_Obj1RelPositionXEst_m : Outport
  VOBJ_Obj1RelVelocityXEst_mps : Outport  Port=2
  VOBJ_Obj1RelAccXEst_mps2 : Outport  Port=3
  VOBJ_Obj1EstValid_flg : Outport  Port=4
  wires:
  VOBJ_Obj1RelPositionXKalF_m/1 -> Switch/1, Compare To Zero/1
  Compare To Zero/1 -> [VOBJ_Obj1EstValid_flg]
  [VOBJ_Obj1EstValid_flg] -> VOBJ_Obj1EstValid_flg/1  "VOBJ_Obj1EstValid_flg"
  [VOBJ_Obj1EstValid_flg] -> Switch/2
  Switch/1 -> VOBJ_Obj1RelPositionXEst_m/1  "VOBJ_Obj1RelPositionXEst_m"
  Constant/1 -> Switch/3
  [VOBJ_Obj1EstValid_flg] -> Switch1/2
  Switch1/1 -> VOBJ_Obj1RelVelocityXEst_mps/1  "VOBJ_Obj1RelVelocityXEst_mps"
  Constant1/1 -> Switch1/3
  [VOBJ_Obj1EstValid_flg] -> Switch2/2
  Switch2/1 -> VOBJ_Obj1RelAccXEst_mps2/1  "VOBJ_Obj1RelAccXEst_mps2"
  Constant2/1 -> Switch2/3
  VOBJ_Obj1RelVelocityXKalF_mps/1 -> Switch1/1
  VOBJ_Obj1RelAccXKalF_mps2/1 -> Switch2/1

== system AEBMIL/OBJ/OBJ/Obj1_RelVelocity_Calculation ==
  VTRCK_Obj1ConfidLevel_enum : Inport
  VTRCK_Obj1PositionX_m : Inport  Port=2
  Compare To Constant2 : simulink/Logic and Bit Operations/Compare To Constant  relop=~=  const=0  OutDataTypeStr=boolean
  DataPass_Obj1 : Subsystem  TreatAsAtomicUnit=on
  Detect Change1 : simulink/Logic and Bit Operations/Detect Change  vinit=0  InputProcessing=Inherited  OutDataTypeStr=boolean
  Detect Decrease : simulink/Logic and Bit Operations/Detect Decrease  vinit=0.0  InputProcessing=Inherited  OutDataTypeStr=boolean
  Detect Increase : simulink/Logic and Bit Operations/Detect Increase  vinit=0.0  InputProcessing=Inherited  OutDataTypeStr=boolean
  Logical Operator3 : Logic  Operator=NOT  AllPortsSameDT=off  OutDataTypeStr=boolean
  Logical Operator4 : Logic  AllPortsSameDT=off  OutDataTypeStr=boolean
  Obj1_RelVelocity_Cal : Subsystem
  SR-Latch : hcu_lib/SR-Latch
  SandH_Obj1 : Subsystem  TreatAsAtomicUnit=on
  Timer1 : Subsystem  TreatAsAtomicUnit=on
  Unit Delay1 : UnitDelay  SampleTime=-1
  VOBJ_Obj1RelVelocityCal_mps : Outport
  wires:
  Obj1_RelVelocity_Cal/1(VOBJ_Obj1RelVelocityCal_mps) -> VOBJ_Obj1RelVelocityCal_mps/1
  Compare To Constant2/1 -> Logical Operator4/2
  Unit Delay1/1 -> Logical Operator3/1
  Logical Operator4/1 -> Timer1/Enable
  Logical Operator3/1 -> Logical Operator4/1
  SandH_Obj1/1(Out1) -> Obj1_RelVelocity_Cal/2(TimeDur_s)
  Timer1/1(Timer (sec)) -> SandH_Obj1/1(In1)
  DataPass_Obj1/1(Out1) -> Obj1_RelVelocity_Cal/1(ObjPositionX_m), Detect Change1/1, Compare To Constant2/1
  Detect Change1/1 -> Unit Delay1/1, SandH_Obj1/Trigger, Obj1_RelVelocity_Cal/Trigger
  VTRCK_Obj1PositionX_m/1 -> DataPass_Obj1/1(In1)
  SR-Latch/1 -> DataPass_Obj1/Enable  "VOBJ_Obj1DataUpdated_flg"
  Detect Increase/1 -> SR-Latch/1
  Detect Decrease/1 -> SR-Latch/2
  VTRCK_Obj1ConfidLevel_enum/1 -> Detect Decrease/1, Detect Increase/1

== system AEBMIL/OBJ/OBJ/Obj2_RelVelocity_Calculation ==
  VTRCK_Obj2ConfidLevel_enum : Inport
  VTRCK_Obj2PositionX_m : Inport  Port=2
  Compare To Constant1 : simulink/Logic and Bit Operations/Compare To Constant  relop=~=  const=0  OutDataTypeStr=boolean
  DataPass_Obj2 : Subsystem  TreatAsAtomicUnit=on
  Detect Change2 : simulink/Logic and Bit Operations/Detect Change  vinit=0  InputProcessing=Inherited  OutDataTypeStr=boolean
  Detect Decrease1 : simulink/Logic and Bit Operations/Detect Decrease  vinit=0.0  InputProcessing=Inherited  OutDataTypeStr=boolean
  Detect Increase1 : simulink/Logic and Bit Operations/Detect Increase  vinit=0.0  InputProcessing=Inherited  OutDataTypeStr=boolean
  Logical Operator1 : Logic  Operator=NOT  AllPortsSameDT=off  OutDataTypeStr=boolean
  Logical Operator2 : Logic  AllPortsSameDT=off  OutDataTypeStr=boolean
  Obj2_RelVelocity_Cal : Subsystem
  SR-Latch1 : hcu_lib/SR-Latch
  SandH_Obj2 : Subsystem  TreatAsAtomicUnit=on
  Timer2 : Subsystem  TreatAsAtomicUnit=on
  Unit Delay2 : UnitDelay  SampleTime=-1
  VOBJ_Obj2RelVelocityCal_mps : Outport
  wires:
  Detect Decrease1/1 -> SR-Latch1/2
  SR-Latch1/1 -> DataPass_Obj2/Enable  "VOBJ_Obj2DataUpdated_flg"
  Logical Operator2/1 -> Timer2/Enable
  SandH_Obj2/1(Out1) -> Obj2_RelVelocity_Cal/2(TimeDur_s)
  Compare To Constant1/1 -> Logical Operator2/2
  VTRCK_Obj2ConfidLevel_enum/1 -> Detect Increase1/1, Detect Decrease1/1
  VTRCK_Obj2PositionX_m/1 -> DataPass_Obj2/1(In1)
  Detect Change2/1 -> Obj2_RelVelocity_Cal/Trigger, SandH_Obj2/Trigger, Unit Delay2/1
  Detect Increase1/1 -> SR-Latch1/1
  DataPass_Obj2/1(Out1) -> Compare To Constant1/1, Detect Change2/1, Obj2_RelVelocity_Cal/1(ObjPositionX_m)
  Obj2_RelVelocity_Cal/1(VOBJ_Obj2RelVelocityCal_mps) -> VOBJ_Obj2RelVelocityCal_mps/1
  Logical Operator1/1 -> Logical Operator2/1
  Timer2/1(Timer (sec)) -> SandH_Obj2/1(In1)
  Unit Delay2/1 -> Logical Operator1/1

== system AEBMIL/OBJ/OBJ/Obj3_RelVelocity_Calculation ==
  VTRCK_Obj3ConfidLevel_enum : Inport
  VTRCK_Obj3PositionX_m : Inport  Port=2
  Compare To Constant3 : simulink/Logic and Bit Operations/Compare To Constant  relop=~=  const=0  OutDataTypeStr=boolean
  DataPass_Obj3 : Subsystem  TreatAsAtomicUnit=on
  Detect Change3 : simulink/Logic and Bit Operations/Detect Change  vinit=0  InputProcessing=Inherited  OutDataTypeStr=boolean
  Detect Decrease2 : simulink/Logic and Bit Operations/Detect Decrease  vinit=0.0  InputProcessing=Inherited  OutDataTypeStr=boolean
  Detect Increase2 : simulink/Logic and Bit Operations/Detect Increase  vinit=0.0  InputProcessing=Inherited  OutDataTypeStr=boolean
  Logical Operator5 : Logic  Operator=NOT  AllPortsSameDT=off  OutDataTypeStr=boolean
  Logical Operator6 : Logic  AllPortsSameDT=off  OutDataTypeStr=boolean
  Obj3_RelVelocity_Cal : Subsystem
  SR-Latch2 : hcu_lib/SR-Latch
  SandH_Obj3 : Subsystem  TreatAsAtomicUnit=on
  Timer3 : Subsystem  TreatAsAtomicUnit=on
  Unit Delay3 : UnitDelay  SampleTime=-1
  VOBJ_Obj3RelVelocityCal_mps : Outport
  wires:
  Detect Change3/1 -> Unit Delay3/1, SandH_Obj3/Trigger, Obj3_RelVelocity_Cal/Trigger
  Compare To Constant3/1 -> Logical Operator6/2
  Logical Operator5/1 -> Logical Operator6/1
  Detect Decrease2/1 -> SR-Latch2/2
  Obj3_RelVelocity_Cal/1(VOBJ_Obj3RelVelocityCal_mps) -> VOBJ_Obj3RelVelocityCal_mps/1
  VTRCK_Obj3ConfidLevel_enum/1 -> Detect Decrease2/1, Detect Increase2/1
  Timer3/1(Timer (sec)) -> SandH_Obj3/1(In1)
  SR-Latch2/1 -> DataPass_Obj3/Enable  "VOBJ_Obj3DataUpdated_flg"
  Detect Increase2/1 -> SR-Latch2/1
  Unit Delay3/1 -> Logical Operator5/1
  DataPass_Obj3/1(Out1) -> Obj3_RelVelocity_Cal/1(ObjPositionX_m), Detect Change3/1, Compare To Constant3/1
  VTRCK_Obj3PositionX_m/1 -> DataPass_Obj3/1(In1)
  SandH_Obj3/1(Out1) -> Obj3_RelVelocity_Cal/2(TimeDur_s)
  Logical Operator6/1 -> Timer3/Enable

== system AEBMIL/OBJ/OBJ/Obj4_RelVelocity_Calculation ==
  VTRCK_Obj4ConfidLevel_enum : Inport
  VTRCK_Obj4PositionX_m : Inport  Port=2
  Compare To Constant4 : simulink/Logic and Bit Operations/Compare To Constant  relop=~=  const=0  OutDataTypeStr=boolean
  DataPass_Obj4 : Subsystem  TreatAsAtomicUnit=on
  Detect Change4 : simulink/Logic and Bit Operations/Detect Change  vinit=0  InputProcessing=Inherited  OutDataTypeStr=boolean
  Detect Decrease3 : simulink/Logic and Bit Operations/Detect Decrease  vinit=0.0  InputProcessing=Inherited  OutDataTypeStr=boolean
  Detect Increase3 : simulink/Logic and Bit Operations/Detect Increase  vinit=0.0  InputProcessing=Inherited  OutDataTypeStr=boolean
  Logical Operator7 : Logic  Operator=NOT  AllPortsSameDT=off  OutDataTypeStr=boolean
  Logical Operator8 : Logic  AllPortsSameDT=off  OutDataTypeStr=boolean
  Obj4_RelVelocity_Cal : Subsystem
  SR-Latch3 : hcu_lib/SR-Latch
  SandH_Obj4 : Subsystem  TreatAsAtomicUnit=on
  Timer4 : Subsystem  TreatAsAtomicUnit=on
  Unit Delay4 : UnitDelay  SampleTime=-1
  VOBJ_Obj4RelVelocityCal_mps : Outport
  wires:
  Logical Operator7/1 -> Logical Operator8/1
  Compare To Constant4/1 -> Logical Operator8/2
  Timer4/1(Timer (sec)) -> SandH_Obj4/1(In1)
  Logical Operator8/1 -> Timer4/Enable
  SandH_Obj4/1(Out1) -> Obj4_RelVelocity_Cal/2(TimeDur_s)
  Unit Delay4/1 -> Logical Operator7/1
  Obj4_RelVelocity_Cal/1(VOBJ_Obj4RelVelocityCal_mps) -> VOBJ_Obj4RelVelocityCal_mps/1
  Detect Change4/1 -> Obj4_RelVelocity_Cal/Trigger, SandH_Obj4/Trigger, Unit Delay4/1
  DataPass_Obj4/1(Out1) -> Compare To Constant4/1, Detect Change4/1, Obj4_RelVelocity_Cal/1(ObjPositionX_m)
  Detect Increase3/1 -> SR-Latch3/1
  VTRCK_Obj4ConfidLevel_enum/1 -> Detect Increase3/1, Detect Decrease3/1
  SR-Latch3/1 -> DataPass_Obj4/Enable  "VOBJ_Obj4DataUpdated_flg"
  VTRCK_Obj4PositionX_m/1 -> DataPass_Obj4/1(In1)
  Detect Decrease3/1 -> SR-Latch3/2

== system AEBMIL/OBJ/OBJ/Obj5_RelVelocity_Calculation ==
  VTRCK_Obj5ConfidLevel_enum : Inport
  VTRCK_Obj5PositionX_m : Inport  Port=2
  Compare To Constant5 : simulink/Logic and Bit Operations/Compare To Constant  relop=~=  const=0  OutDataTypeStr=boolean
  DataPass_Obj5 : Subsystem  TreatAsAtomicUnit=on
  Detect Change5 : simulink/Logic and Bit Operations/Detect Change  vinit=0  InputProcessing=Inherited  OutDataTypeStr=boolean
  Detect Decrease4 : simulink/Logic and Bit Operations/Detect Decrease  vinit=0.0  InputProcessing=Inherited  OutDataTypeStr=boolean
  Detect Increase4 : simulink/Logic and Bit Operations/Detect Increase  vinit=0.0  InputProcessing=Inherited  OutDataTypeStr=boolean
  Logical Operator10 : Logic  AllPortsSameDT=off  OutDataTypeStr=boolean
  Logical Operator9 : Logic  Operator=NOT  AllPortsSameDT=off  OutDataTypeStr=boolean
  Obj5_RelVelocity_Cal : Subsystem
  SR-Latch4 : hcu_lib/SR-Latch
  SandH_Obj5 : Subsystem  TreatAsAtomicUnit=on
  Timer5 : Subsystem  TreatAsAtomicUnit=on
  Unit Delay5 : UnitDelay  SampleTime=-1
  VOBJ_Obj5RelVelocityCal_mps : Outport
  wires:
  Obj5_RelVelocity_Cal/1(VOBJ_Obj5RelVelocityCal_mps) -> VOBJ_Obj5RelVelocityCal_mps/1
  Unit Delay5/1 -> Logical Operator9/1
  Compare To Constant5/1 -> Logical Operator10/2
  Logical Operator10/1 -> Timer5/Enable
  Logical Operator9/1 -> Logical Operator10/1
  SandH_Obj5/1(Out1) -> Obj5_RelVelocity_Cal/2(TimeDur_s)
  Timer5/1(Timer (sec)) -> SandH_Obj5/1(In1)
  Detect Decrease4/1 -> SR-Latch4/2
  Detect Increase4/1 -> SR-Latch4/1
  VTRCK_Obj5ConfidLevel_enum/1 -> Detect Decrease4/1, Detect Increase4/1
  Detect Change5/1 -> Unit Delay5/1, SandH_Obj5/Trigger, Obj5_RelVelocity_Cal/Trigger
  DataPass_Obj5/1(Out1) -> Obj5_RelVelocity_Cal/1(ObjPositionX_m), Detect Change5/1, Compare To Constant5/1
  SR-Latch4/1 -> DataPass_Obj5/Enable  "VOBJ_Obj5DataUpdated_flg"
  VTRCK_Obj5PositionX_m/1 -> DataPass_Obj5/1(In1)

== system AEBMIL/OBJ/OBJ/Trigger signal generator ==
  Constant3 : Constant  Value=KOBJ_KalmanFilterCalRate_s
  trigger signal generator : Subsystem  TreatAsAtomicUnit=on
  Trigger_signal : Outport
  wires:
  trigger signal generator/1(Trigger_signal) -> Trigger_signal/1
  Constant3/1 -> trigger signal generator/1(Time_dur [s])

== system AEBMIL/OBJ/OBJ/Trigger signal generator1 ==
  Constant3 : Constant  Value=KOBJ_VehAccCalRate_s
  trigger signal generator : Subsystem  TreatAsAtomicUnit=on
  Trigger_signal : Outport
  wires:
  trigger signal generator/1(Trigger_signal) -> Trigger_signal/1
  Constant3/1 -> trigger signal generator/1(Time_dur [s])

== system AEBMIL/OBJ/OBJ/Vehicle Acceleration Calculation ==
  note: m/s^2
  note: m/s
  note: km/h
  In1 : Inport
  Trigger : TriggerPort
  Constant2 : Constant  Value=KOBJ_VehAccCalRate_s
  Constant3 : Constant  Value=KOBJ_VehAccCalRate_s
  Constant4 : Constant  Value=KOBJ_VehAccFltConst_s
  Divide : Product  Inputs=*/
  Gain : Gain  Gain=1000/3600
  Sum : Sum  Inputs=+-
  Unit Delay : UnitDelay  SampleTime=-1
  signal_filter : Subsystem
  VOBJ_VehAcc_mps2 : Outport
  wires:
  signal_filter/1(raw_input_filt) -> VOBJ_VehAcc_mps2/1  "VOBJ_VehAcc_mps2"
  Constant3/1 -> Divide/2
  Gain/1 -> Divide/1
  Sum/1 -> Gain/1
  Unit Delay/1 -> Sum/2
  In1/1 -> Sum/1, Unit Delay/1
  Constant2/1 -> signal_filter/3(Ts)
  Constant4/1 -> signal_filter/2(Tc)
  Divide/1 -> signal_filter/1(raw_input)  "VOBJ_VehAcclUnFlt_mps2"

== system AEBMIL/OBJ/model_info/EmptySubsystem ==

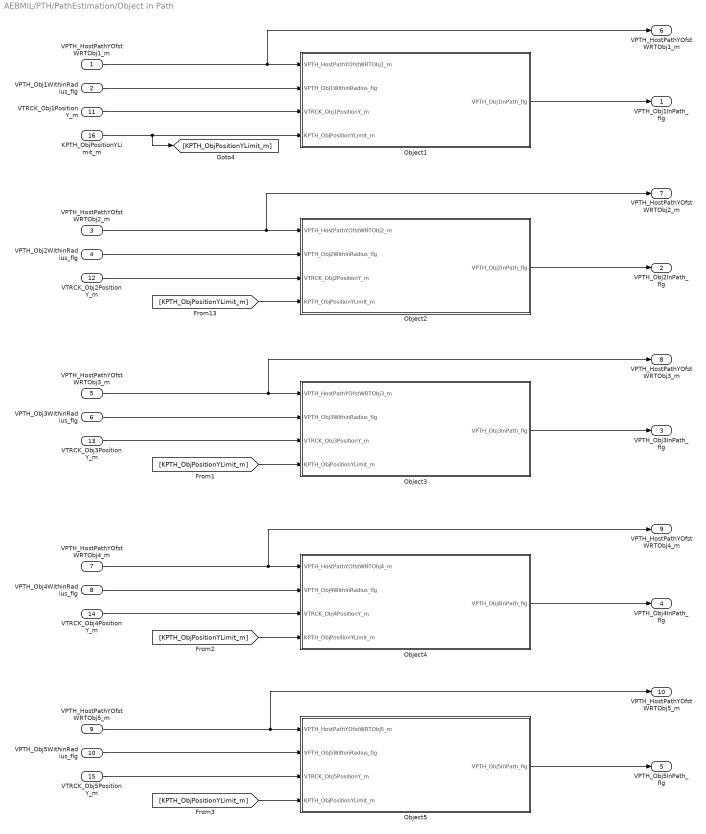
== system AEBMIL/PTH/PathEstimation/Object in Path ==
  VPTH_HostPathYOfstWRTObj1_m : Inport
  VPTH_Obj1WithinRadius_flg : Inport  Port=2
  VPTH_HostPathYOfstWRTObj2_m : Inport  Port=3
  VPTH_Obj2WithinRadius_flg : Inport  Port=4
  VPTH_HostPathYOfstWRTObj3_m : Inport  Port=5
  VPTH_Obj3WithinRadius_flg : Inport  Port=6
  VPTH_HostPathYOfstWRTObj4_m : Inport  Port=7
  VPTH_Obj4WithinRadius_flg : Inport  Port=8
  VPTH_HostPathYOfstWRTObj5_m : Inport  Port=9
  VPTH_Obj5WithinRadius_flg : Inport  Port=10
  VTRCK_Obj1PositionY_m : Inport  Port=11
  VTRCK_Obj2PositionY_m : Inport  Port=12
  VTRCK_Obj3PositionY_m : Inport  Port=13
  VTRCK_Obj4PositionY_m : Inport  Port=14
  VTRCK_Obj5PositionY_m : Inport  Port=15
  KPTH_ObjPositionYLimit_m : Inport  Port=16
  Object1 : Subsystem
  Object2 : Subsystem
  Object3 : Subsystem
  Object4 : Subsystem
  Object5 : Subsystem
  VPTH_Obj1InPath_flg : Outport
  VPTH_Obj2InPath_flg : Outport  Port=2
  VPTH_Obj3InPath_flg : Outport  Port=3
  VPTH_Obj4InPath_flg : Outport  Port=4
  VPTH_Obj5InPath_flg : Outport  Port=5
  "VPTH_HostPathYOfstWRTObj1_m " : Outport  Port=6
  "VPTH_HostPathYOfstWRTObj2_m " : Outport  Port=7
  "VPTH_HostPathYOfstWRTObj3_m " : Outport  Port=8
  "VPTH_HostPathYOfstWRTObj4_m " : Outport  Port=9
  "VPTH_HostPathYOfstWRTObj5_m " : Outport  Port=10
  wires:
  [KPTH_ObjPositionYLimit_m] -> Object5/4(KPTH_ObjPositionYLimit_m)
  Object5/1(VPTH_Obj5InPath_flg) -> VPTH_Obj5InPath_flg/1
  VTRCK_Obj5PositionY_m/1 -> Object5/3(VTRCK_Obj5PositionY_m)
  VPTH_Obj5WithinRadius_flg/1 -> Object5/2(VPTH_Obj5WithinRadius_flg)
  VPTH_HostPathYOfstWRTObj5_m/1 -> Object5/1(VPTH_HostPathYOfstWRTObj5_m), "VPTH_HostPathYOfstWRTObj5_m "/1
  [KPTH_ObjPositionYLimit_m] -> Object4/4(KPTH_ObjPositionYLimit_m)
  Object4/1(VPTH_Obj4InPath_flg) -> VPTH_Obj4InPath_flg/1
  VTRCK_Obj4PositionY_m/1 -> Object4/3(VTRCK_Obj4PositionY_m)
  VPTH_Obj4WithinRadius_flg/1 -> Object4/2(VPTH_Obj4WithinRadius_flg)
  VPTH_HostPathYOfstWRTObj4_m/1 -> Object4/1(VPTH_HostPathYOfstWRTObj4_m), "VPTH_HostPathYOfstWRTObj4_m "/1
  [KPTH_ObjPositionYLimit_m] -> Object3/4(KPTH_ObjPositionYLimit_m)
  Object3/1(VPTH_Obj3InPath_flg) -> VPTH_Obj3InPath_flg/1
  VTRCK_Obj3PositionY_m/1 -> Object3/3(VTRCK_Obj3PositionY_m)
  VPTH_Obj3WithinRadius_flg/1 -> Object3/2(VPTH_Obj3WithinRadius_flg)
  VPTH_HostPathYOfstWRTObj3_m/1 -> Object3/1(VPTH_HostPathYOfstWRTObj3_m), "VPTH_HostPathYOfstWRTObj3_m "/1
  [KPTH_ObjPositionYLimit_m] -> Object2/4(KPTH_ObjPositionYLimit_m)
  Object2/1(VPTH_Obj2InPath_flg) -> VPTH_Obj2InPath_flg/1
  VTRCK_Obj2PositionY_m/1 -> Object2/3(VTRCK_Obj2PositionY_m)
  VPTH_Obj2WithinRadius_flg/1 -> Object2/2(VPTH_Obj2WithinRadius_flg)
  VPTH_HostPathYOfstWRTObj2_m/1 -> Object2/1(VPTH_HostPathYOfstWRTObj2_m), "VPTH_HostPathYOfstWRTObj2_m "/1
  Object1/1(VPTH_Obj1InPath_flg) -> VPTH_Obj1InPath_flg/1
  KPTH_ObjPositionYLimit_m/1 -> Object1/4(KPTH_ObjPositionYLimit_m), [KPTH_ObjPositionYLimit_m]
  VTRCK_Obj1PositionY_m/1 -> Object1/3(VTRCK_Obj1PositionY_m)
  VPTH_Obj1WithinRadius_flg/1 -> Object1/2(VPTH_Obj1WithinRadius_flg)
  VPTH_HostPathYOfstWRTObj1_m/1 -> Object1/1(VPTH_HostPathYOfstWRTObj1_m), "VPTH_HostPathYOfstWRTObj1_m "/1

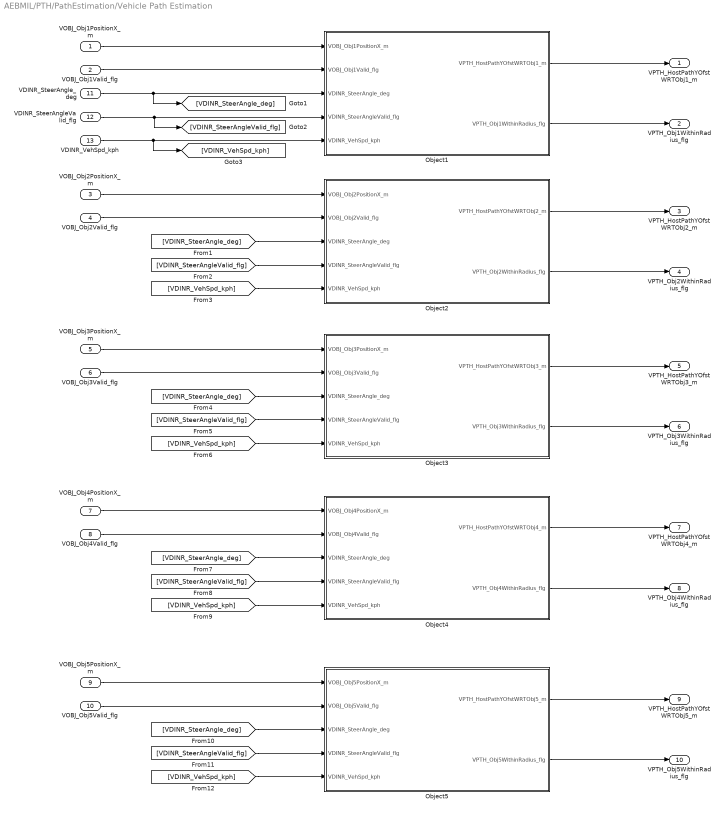
== system AEBMIL/PTH/PathEstimation/Vehicle Path Estimation ==
  VOBJ_Obj1PositionX_m : Inport
  VOBJ_Obj1Valid_flg : Inport  Port=2
  VOBJ_Obj2PositionX_m : Inport  Port=3
  VOBJ_Obj2Valid_flg : Inport  Port=4
  VOBJ_Obj3PositionX_m : Inport  Port=5
  VOBJ_Obj3Valid_flg : Inport  Port=6
  VOBJ_Obj4PositionX_m : Inport  Port=7
  VOBJ_Obj4Valid_flg : Inport  Port=8
  VOBJ_Obj5PositionX_m : Inport  Port=9
  VOBJ_Obj5Valid_flg : Inport  Port=10
  VDINR_SteerAngle_deg : Inport  Port=11
  VDINR_SteerAngleValid_flg : Inport  Port=12
  VDINR_VehSpd_kph : Inport  Port=13
  Object1 : Subsystem
  Object2 : Subsystem
  Object3 : Subsystem
  Object4 : Subsystem
  Object5 : Subsystem
  VPTH_HostPathYOfstWRTObj1_m : Outport
  VPTH_Obj1WithinRadius_flg : Outport  Port=2
  VPTH_HostPathYOfstWRTObj2_m : Outport  Port=3
  VPTH_Obj2WithinRadius_flg : Outport  Port=4
  VPTH_HostPathYOfstWRTObj3_m : Outport  Port=5
  VPTH_Obj3WithinRadius_flg : Outport  Port=6
  VPTH_HostPathYOfstWRTObj4_m : Outport  Port=7
  VPTH_Obj4WithinRadius_flg : Outport  Port=8
  VPTH_HostPathYOfstWRTObj5_m : Outport  Port=9
  VPTH_Obj5WithinRadius_flg : Outport  Port=10
  wires:
  VOBJ_Obj5Valid_flg/1 -> Object5/2(VOBJ_Obj5Valid_flg)
  VOBJ_Obj4Valid_flg/1 -> Object4/2(VOBJ_Obj4Valid_flg)
  VOBJ_Obj3Valid_flg/1 -> Object3/2(VOBJ_Obj3Valid_flg)
  VOBJ_Obj2Valid_flg/1 -> Object2/2(VOBJ_Obj2Valid_flg)
  VOBJ_Obj1Valid_flg/1 -> Object1/2(VOBJ_Obj1Valid_flg)
  [VDINR_VehSpd_kph] -> Object5/5(VDINR_VehSpd_kph)
  [VDINR_SteerAngle_deg] -> Object5/3(VDINR_SteerAngle_deg)
  [VDINR_SteerAngleValid_flg] -> Object5/4(VDINR_SteerAngleValid_flg)
  Object5/2(VPTH_Obj5WithinRadius_flg) -> VPTH_Obj5WithinRadius_flg/1
  Object5/1(VPTH_HostPathYOfstWRTObj5_m) -> VPTH_HostPathYOfstWRTObj5_m/1
  VOBJ_Obj5PositionX_m/1 -> Object5/1(VOBJ_Obj5PositionX_m)
  [VDINR_VehSpd_kph] -> Object4/5(VDINR_VehSpd_kph)
  [VDINR_SteerAngleValid_flg] -> Object4/4(VDINR_SteerAngleValid_flg)
  [VDINR_SteerAngle_deg] -> Object4/3(VDINR_SteerAngle_deg)
  Object4/2(VPTH_Obj4WithinRadius_flg) -> VPTH_Obj4WithinRadius_flg/1
  Object4/1(VPTH_HostPathYOfstWRTObj4_m) -> VPTH_HostPathYOfstWRTObj4_m/1
  VOBJ_Obj4PositionX_m/1 -> Object4/1(VOBJ_Obj4PositionX_m)
  [VDINR_SteerAngle_deg] -> Object3/3(VDINR_SteerAngle_deg)
  [VDINR_SteerAngleValid_flg] -> Object3/4(VDINR_SteerAngleValid_flg)
  [VDINR_VehSpd_kph] -> Object3/5(VDINR_VehSpd_kph)
  Object3/2(VPTH_Obj3WithinRadius_flg) -> VPTH_Obj3WithinRadius_flg/1
  Object3/1(VPTH_HostPathYOfstWRTObj3_m) -> VPTH_HostPathYOfstWRTObj3_m/1
  VOBJ_Obj3PositionX_m/1 -> Object3/1(VOBJ_Obj3PositionX_m)
  [VDINR_VehSpd_kph] -> Object2/5(VDINR_VehSpd_kph)
  [VDINR_SteerAngleValid_flg] -> Object2/4(VDINR_SteerAngleValid_flg)
  [VDINR_SteerAngle_deg] -> Object2/3(VDINR_SteerAngle_deg)
  Object2/2(VPTH_Obj2WithinRadius_flg) -> VPTH_Obj2WithinRadius_flg/1
  Object2/1(VPTH_HostPathYOfstWRTObj2_m) -> VPTH_HostPathYOfstWRTObj2_m/1
  VOBJ_Obj2PositionX_m/1 -> Object2/1(VOBJ_Obj2PositionX_m)
  Object1/2(VPTH_Obj1WithinRadius_flg) -> VPTH_Obj1WithinRadius_flg/1
  Object1/1(VPTH_HostPathYOfstWRTObj1_m) -> VPTH_HostPathYOfstWRTObj1_m/1
  VDINR_VehSpd_kph/1 -> Object1/5(VDINR_VehSpd_kph), [VDINR_VehSpd_kph]
  VDINR_SteerAngleValid_flg/1 -> Object1/4(VDINR_SteerAngleValid_flg), [VDINR_SteerAngleValid_flg]
  VDINR_SteerAngle_deg/1 -> Object1/3(VDINR_SteerAngle_deg), [VDINR_SteerAngle_deg]
  VOBJ_Obj1PositionX_m/1 -> Object1/1(VOBJ_Obj1PositionX_m)

== system AEBMIL/PTH/model_info/EmptySubsystem ==

== system AEBMIL/TTC/model_info/EmptySubsystem ==
